simulink model "test2_stateflow_v2"  (R2017b)
settings: Solver=VariableStepAuto  StartTime=0.0  StopTime=inf  RelTol=1e-3
settings Model: Creator=Bijan  LastModifiedBy=Bijan

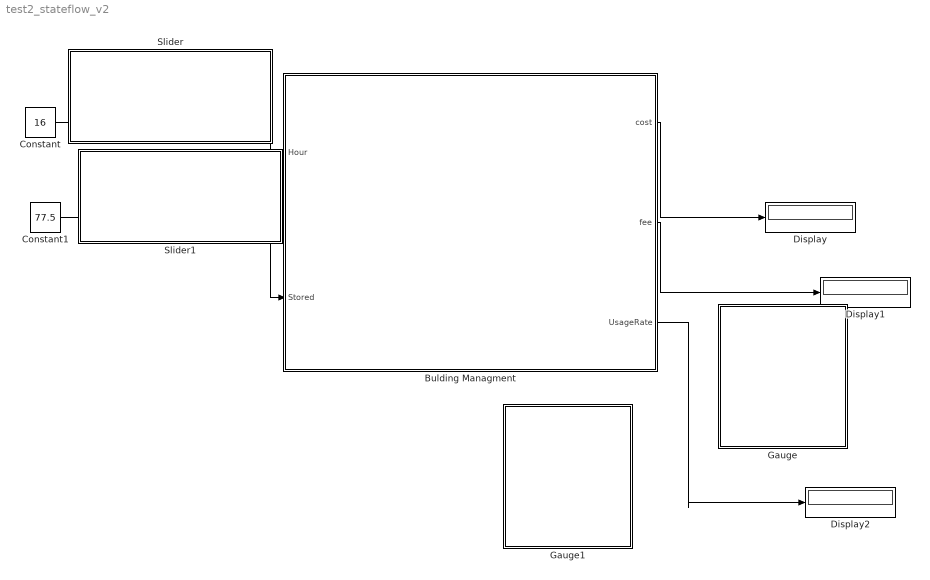
== system test2_stateflow_v2 ==
  Bulding Managment : Stateflow chart  TreatAsAtomicUnit=on
  Constant : Constant  Value=16
  Constant1 : Constant  Value=77.5
  Display : Display
  Display1 : Display
  Display2 : Display
  Gauge : Subsystem  DialogController=hmiCreateDDGDialog  IsWebBlock=on  mask(MWDashboardBlock){webBlockId=8d7f4243-faa0-4b05-b0e1-7aa234a6f188, webBlockType=circulargauge, ShowInLibBrowser=on, ShowInitialText=on, HMISrcModelName=test2_stateflow_v2}
      mask prompts: webBlockId "WebBlock Id"; webBlockType "WebBlock Type"; HMISrcModelName "Source Model"
      mask help: SimulinkHMI:dialogs:CircularGaugeDialogDesc
      mask Help: helpview([docroot '/mapfiles/simulink.map'], 'hmi_gauge')
      mask Display:
      | if strcmp(get_param(bdroot(gcb),'BlockDiagramType'), 'library')
      |     image([(matlabroot) '/toolbox/simulink/hmi/icons/CircularGauge.png']);
      | end
  Gauge1 : Subsystem  DialogController=hmiCreateDDGDialog  IsWebBlock=on  mask(MWDashboardBlock){webBlockId=309a1f03-f6f9-473e-8be3-aecc213c69dc, webBlockType=circulargauge, ShowInLibBrowser=on, ShowInitialText=on, HMISrcModelName=test2_stateflow_v2}
      mask prompts: webBlockId "WebBlock Id"; webBlockType "WebBlock Type"; HMISrcModelName "Source Model"
      mask help: SimulinkHMI:dialogs:CircularGaugeDialogDesc
      mask Help: helpview([docroot '/mapfiles/simulink.map'], 'hmi_gauge')
      mask Display:
      | if strcmp(get_param(bdroot(gcb),'BlockDiagramType'), 'library')
      |     image([(matlabroot) '/toolbox/simulink/hmi/icons/CircularGauge.png']);
      | end
  Slider : Subsystem  DialogController=hmiCreateDDGDialog  IsWebBlock=on  mask(MWDashboardBlock){webBlockId=a443525b-c956-4c8b-a501-0a83e762846b, webBlockType=slider, ShowInLibBrowser=on, ShowInitialText=on, HMISrcModelName=test2_stateflow_v2}
      mask prompts: webBlockId "WebBlock Id"; webBlockType "WebBlock Type"; HMISrcModelName "Source Model"
      mask help: SimulinkHMI:dialogs:SliderDialogDesc
      mask Help: helpview([docroot '/mapfiles/simulink.map'], 'hmi_slider')
      mask Display:
      | if strcmp(get_param(bdroot(gcb),'BlockDiagramType'), 'library')
      |     image([(matlabroot) '/toolbox/simulink/hmi/icons/Slider.png']);
      | end
  Slider1 : Subsystem  DialogController=hmiCreateDDGDialog  IsWebBlock=on  mask(MWDashboardBlock){webBlockId=6981fd38-2443-492a-a3b7-98ef9a373d3b, webBlockType=slider, ShowInLibBrowser=on, ShowInitialText=on, HMISrcModelName=test2_stateflow_v2}
      mask prompts: webBlockId "WebBlock Id"; webBlockType "WebBlock Type"; HMISrcModelName "Source Model"
      mask help: SimulinkHMI:dialogs:SliderDialogDesc
      mask Help: helpview([docroot '/mapfiles/simulink.map'], 'hmi_slider')
      mask Display:
      | if strcmp(get_param(bdroot(gcb),'BlockDiagramType'), 'library')
      |     image([(matlabroot) '/toolbox/simulink/hmi/icons/Slider.png']);
      | end
  wires:
  Constant/1 -> Bulding Managment/1(Hour)
  Constant1/1 -> Bulding Managment/2(Stored)
  Bulding Managment/1(cost) -> Display/1
  Bulding Managment/2(fee) -> Display1/1
  Bulding Managment/3(UsageRate) -> Display2/1

== system test2_stateflow_v2/Gauge ==

== system test2_stateflow_v2/Gauge1 ==

== system test2_stateflow_v2/Slider ==

== system test2_stateflow_v2/Slider1 ==

== stateflow chart test2_stateflow_v2/Bulding Managment ==
  state Time [parallel]
    settings: executionOrder=1
    state OffPeak
    state Peak
    (default) -> OffPeak
    OffPeak -> Peak : [Hour>12 && Hour<18]
    Peak -> OffPeak : [Hour>18 || Hour<12]
  state EnergyManager [parallel]
    settings: executionOrder=2
    state Used_Battery
      entry: UsageRate=200
      during: UsageRate=UsageRate-0.001
      fee=0
      exit:UsageRate=UsageRate
    state Used_Grid
      (default) -> (junction 13)
      Used_Grid -> (junction 13) [order 1]
      (junction 13) -> (junction 15) [order 1] : [in(Time.Peak)]
      (junction 13) -> (junction 17) [order 2] : {fee=10,
          | cost=cost+10}
      (junction 15) -> (junction 16) : {fee=15,cost=cost+15}
      (junction 16) -> (junction 17)
    (default) -> Used_Grid : {cost=0,fee=0}
    Used_Grid -> Used_Battery [order 1] : [Stored>50]
    Used_Battery -> Used_Grid : [Stored<50]
  data: data local; Hour input; Stored input; cost output; fee output; UsageRate output
